simulink model "wrench_observer_R2016b"  (R2016b)
settings: Solver=VariableStepAuto  StartTime=0.0  StopTime=0.75  RelTol=1e-3
InitFcn:
  | %x_k1 = 0.00001*ones(36,1); % initialisation with initial state uncertainity
  | %P_k1 = 0.00001*ones(36); % initialisation with initial state uncertainity
values from neighbouring files (symbols this model uses):
  a_noise = 0    [parameter.m]
  alpha1 = pi/2    (= 1.57079632679)    [parameter.m]
  alpha2 = 0    [parameter.m]
  alpha3 = 0    [parameter.m]
  angular_noise = 0    [parameter.m]
  g = 9.81    [parameter.m]
  K_f_comm = 1    [parameter.m]
  K_I = [500*eye(3), zeros(3), zeros(3) ... (first row only)    [parameter.m]
  K_tau_comm = 1    [parameter.m]
  K_tau_man_comm = 1    [parameter.m]
  m = 3.9    [parameter.m]
  m_l1 = 0.3    [parameter.m]
  m_l2 = 0.35    [parameter.m]
  m_l3 = 0.35    [parameter.m]
  N_m = 1*diag([(p_noise/(3*noise_factor))^2 (p_noise/(3*noise_factor))^2 (p_noise/(3*noise_factor))^2 (a_noise/(3*noise_factor))^2 (a_noise/(3*noise_factor))^2 (a_noise/(3*noise_factor))^2 (angular_noise/(3*noise_factor))^2 (angular_noise/(3*noise_factor))^2 (angular_noise/(3*noise_factor))^2 (omega_noise/(3*noise_factor))^2 (omega_noise/(3*noise_factor))^2 (omega_noise/(3*noise_factor))^2 (theta_noise/( ...(+272 chars)    [parameter.m]
  N_p = diag(noise_factor_EKF)    [parameter.m]
  omega_dot_noise = 0    [parameter.m]
  omega_noise = 0    [parameter.m]
  p_L1_l1 = [p_L1_x_l1 p_L1_y_l1 p_L1_z_l1]'    [parameter.m]
  p_L2_l2 = [p_L2_x_l2 p_L2_y_l2 p_L2_z_l2]'    [parameter.m]
  p_L3_l3 = [p_L3_x_l3 p_L3_y_l3 p_L3_z_l3]'    [parameter.m]
  p_noise = 0    [parameter.m]
  R_B_L0 = [1 0 0;0 1 0; 0 0 1]    [parameter.m]
  T_delay = 0    [parameter.m]
  T_dis = 0.01    [parameter.m]
  theta_dot_dot_noise = 0    [parameter.m]
  theta_dot_noise = 0    [parameter.m]
  theta_noise = 0    [parameter.m]
  Ts = 1/250    (= 0.004)    [parameter.m]
  v_noise = 0    [parameter.m]
libraries: simulink x9, dspstat3 x2, dspinverses x1
(part 2 of 5)

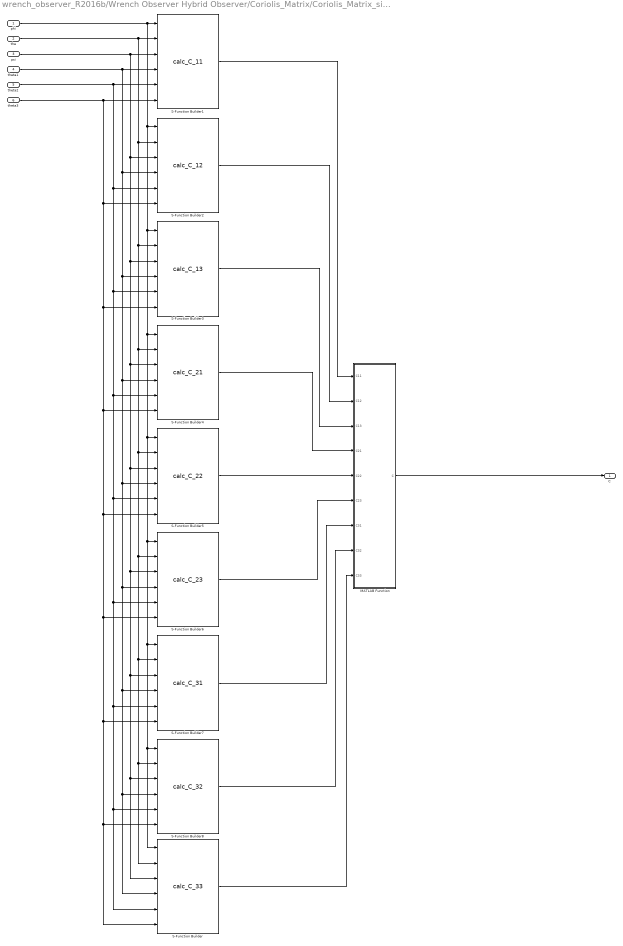
== system wrench_observer_R2016b/Wrench Observer Hybrid Observer/Coriolis_Matrix/Coriolis_Matrix_simplified ==
  phi : Inport
  the : Inport  Port=2
  psi : Inport  Port=3
  theta1 : Inport  Port=4
  theta2 : Inport  Port=5
  theta3 : Inport  Port=6
  MATLAB Function : MATLAB Function  TreatAsAtomicUnit=on
  S-Function Builder : S-Function  InitFcn=try, set_param(gcb,'FunctionName','calc_C_33'), end  FunctionName=calc_C_33  SFunctionModules=calc_C_33_wrapper C_num_simp_33 C_num_simp_33_initialize C_num_simp_33_terminate rt_nonfinite rtGetInf rtGetNaN  SFunctionDeploymentMode=off  EnableBusSupport=off  mask(S-Function Builder){}
      mask help: Simulink:masks:SFunctionBuilder_MD
      mask init: same as wrench_observer_R2016b/Motion Equations with Manipulator /Inertia_Matrix/S-Function Builder
      settings: CopyFcn=set_param(gcbh,'LinkStatus','none')  PreSaveFcn=try, set_param(gcb,'FunctionName','calc_C_33'), end  OpenFcn=sfunctionwizard(gcbh)
      mask Display: plot(val(:,1),val(:,2)),disp(sys), port_label('input',1,'phi'), port_label('input',2,'the'), port_label('input',3,'psi'), port_label('input',4,'theta1'), port_label('input',5,'theta2'), port_label('input',6,'theta3'), port_label('output',1,'C_33')
  S-Function Builder1 : S-Function  InitFcn=try, set_param(gcb,'FunctionName','calc_C_11'), end  FunctionName=calc_C_11  SFunctionModules=calc_C_11_wrapper C_num_simp_11 C_num_simp_11_initialize C_num_simp_11_terminate  SFunctionDeploymentMode=off  EnableBusSupport=off  mask(S-Function Builder){}
      mask help: Simulink:masks:SFunctionBuilder_MD
      mask init: same as wrench_observer_R2016b/Motion Equations with Manipulator /Inertia_Matrix/S-Function Builder
      settings: CopyFcn=set_param(gcbh,'LinkStatus','none')  PreSaveFcn=try, set_param(gcb,'FunctionName','calc_C_11'), end  OpenFcn=sfunctionwizard(gcbh)
      mask Display: plot(val(:,1),val(:,2)),disp(sys), port_label('input',1,'phi'), port_label('input',2,'the'), port_label('input',3,'psi'), port_label('input',4,'theta1'), port_label('input',5,'theta2'), port_label('input',6,'theta3'), port_label('output',1,'C_11')
  S-Function Builder2 : S-Function  InitFcn=try, set_param(gcb,'FunctionName','calc_C_12'), end  FunctionName=calc_C_12  SFunctionModules=calc_C_12_wrapper C_num_simp_12 C_num_simp_12_initialize C_num_simp_12_terminate  SFunctionDeploymentMode=off  EnableBusSupport=off  mask(S-Function Builder){}
      mask help: Simulink:masks:SFunctionBuilder_MD
      mask init: same as wrench_observer_R2016b/Motion Equations with Manipulator /Inertia_Matrix/S-Function Builder
      settings: CopyFcn=set_param(gcbh,'LinkStatus','none')  PreSaveFcn=try, set_param(gcb,'FunctionName','calc_C_12'), end  OpenFcn=sfunctionwizard(gcbh)
      mask Display: plot(val(:,1),val(:,2)),disp(sys), port_label('input',1,'phi'), port_label('input',2,'the'), port_label('input',3,'psi'), port_label('input',4,'theta1'), port_label('input',5,'theta2'), port_label('input',6,'theta3'), port_label('output',1,'C_12')
  S-Function Builder3 : S-Function  InitFcn=try, set_param(gcb,'FunctionName','calc_C_13'), end  FunctionName=calc_C_13  SFunctionModules=calc_C_13_wrapper C_num_simp_13 C_num_simp_13_initialize C_num_simp_13_terminate  SFunctionDeploymentMode=off  EnableBusSupport=off  mask(S-Function Builder){}
      mask help: Simulink:masks:SFunctionBuilder_MD
      mask init: same as wrench_observer_R2016b/Motion Equations with Manipulator /Inertia_Matrix/S-Function Builder
      settings: CopyFcn=set_param(gcbh,'LinkStatus','none')  PreSaveFcn=try, set_param(gcb,'FunctionName','calc_C_13'), end  OpenFcn=sfunctionwizard(gcbh)
      mask Display: plot(val(:,1),val(:,2)),disp(sys), port_label('input',1,'phi'), port_label('input',2,'the'), port_label('input',3,'psi'), port_label('input',4,'theta1'), port_label('input',5,'theta2'), port_label('input',6,'theta3'), port_label('output',1,'C_13')
  S-Function Builder4 : S-Function  InitFcn=try, set_param(gcb,'FunctionName','calc_C_21'), end  FunctionName=calc_C_21  SFunctionModules=calc_C_21_wrapper C_num_simp_21 C_num_simp_21_initialize C_num_simp_21_terminate  SFunctionDeploymentMode=off  EnableBusSupport=off  mask(S-Function Builder){}
      mask help: Simulink:masks:SFunctionBuilder_MD
      mask init: same as wrench_observer_R2016b/Motion Equations with Manipulator /Inertia_Matrix/S-Function Builder
      settings: CopyFcn=set_param(gcbh,'LinkStatus','none')  PreSaveFcn=try, set_param(gcb,'FunctionName','calc_C_21'), end  OpenFcn=sfunctionwizard(gcbh)
      mask Display: plot(val(:,1),val(:,2)),disp(sys), port_label('input',1,'phi'), port_label('input',2,'the'), port_label('input',3,'psi'), port_label('input',4,'theta1'), port_label('input',5,'theta2'), port_label('input',6,'theta3'), port_label('output',1,'C_21')
  S-Function Builder5 : S-Function  InitFcn=try, set_param(gcb,'FunctionName','calc_C_22'), end  FunctionName=calc_C_22  SFunctionModules=calc_C_22_wrapper C_num_simp_22 C_num_simp_22_initialize C_num_simp_22_terminate rt_nonfinite rtGetInf rtGetNaN  SFunctionDeploymentMode=off  EnableBusSupport=off  mask(S-Function Builder){}
      mask help: Simulink:masks:SFunctionBuilder_MD
      mask init: same as wrench_observer_R2016b/Motion Equations with Manipulator /Inertia_Matrix/S-Function Builder
      settings: CopyFcn=set_param(gcbh,'LinkStatus','none')  PreSaveFcn=try, set_param(gcb,'FunctionName','calc_C_22'), end  OpenFcn=sfunctionwizard(gcbh)
      mask Display: plot(val(:,1),val(:,2)),disp(sys), port_label('input',1,'phi'), port_label('input',2,'the'), port_label('input',3,'psi'), port_label('input',4,'theta1'), port_label('input',5,'theta2'), port_label('input',6,'theta3'), port_label('output',1,'C_22')
  S-Function Builder6 : S-Function  InitFcn=try, set_param(gcb,'FunctionName','calc_C_23'), end  FunctionName=calc_C_23  SFunctionModules=calc_C_23_wrapper C_num_simp_23 C_num_simp_23_initialize C_num_simp_23_terminate rt_nonfinite rtGetInf rtGetNaN  SFunctionDeploymentMode=off  EnableBusSupport=off  mask(S-Function Builder){}
      mask help: Simulink:masks:SFunctionBuilder_MD
      mask init: same as wrench_observer_R2016b/Motion Equations with Manipulator /Inertia_Matrix/S-Function Builder
      settings: CopyFcn=set_param(gcbh,'LinkStatus','none')  PreSaveFcn=try, set_param(gcb,'FunctionName','calc_C_23'), end  OpenFcn=sfunctionwizard(gcbh)
      mask Display: plot(val(:,1),val(:,2)),disp(sys), port_label('input',1,'phi'), port_label('input',2,'the'), port_label('input',3,'psi'), port_label('input',4,'theta1'), port_label('input',5,'theta2'), port_label('input',6,'theta3'), port_label('output',1,'C_23')
  S-Function Builder7 : S-Function  InitFcn=try, set_param(gcb,'FunctionName','calc_C_31'), end  FunctionName=calc_C_31  SFunctionModules=calc_C_31_wrapper C_num_simp_31 C_num_simp_31_initialize C_num_simp_31_terminate  SFunctionDeploymentMode=off  EnableBusSupport=off  mask(S-Function Builder){}
      mask help: Simulink:masks:SFunctionBuilder_MD
      mask init: same as wrench_observer_R2016b/Motion Equations with Manipulator /Inertia_Matrix/S-Function Builder
      settings: CopyFcn=set_param(gcbh,'LinkStatus','none')  PreSaveFcn=try, set_param(gcb,'FunctionName','calc_C_31'), end  OpenFcn=sfunctionwizard(gcbh)
      mask Display: plot(val(:,1),val(:,2)),disp(sys), port_label('input',1,'phi'), port_label('input',2,'the'), port_label('input',3,'psi'), port_label('input',4,'theta1'), port_label('input',5,'theta2'), port_label('input',6,'theta3'), port_label('output',1,'C_31')
  S-Function Builder8 : S-Function  InitFcn=try, set_param(gcb,'FunctionName','calc_C_32'), end  FunctionName=calc_C_32  SFunctionModules=calc_C_32_wrapper C_num_simp_32 C_num_simp_32_initialize C_num_simp_32_terminate rt_nonfinite rtGetInf rtGetNaN  SFunctionDeploymentMode=off  EnableBusSupport=off  mask(S-Function Builder){}
      mask help: Simulink:masks:SFunctionBuilder_MD
      mask init: same as wrench_observer_R2016b/Motion Equations with Manipulator /Inertia_Matrix/S-Function Builder
      settings: CopyFcn=set_param(gcbh,'LinkStatus','none')  PreSaveFcn=try, set_param(gcb,'FunctionName','calc_C_32'), end  OpenFcn=sfunctionwizard(gcbh)
      mask Display: plot(val(:,1),val(:,2)),disp(sys), port_label('input',1,'phi'), port_label('input',2,'the'), port_label('input',3,'psi'), port_label('input',4,'theta1'), port_label('input',5,'theta2'), port_label('input',6,'theta3'), port_label('output',1,'C_32')
  C : Outport
  wires:
  S-Function Builder5/1 -> MATLAB Function/5(C22)
  theta2/1 -> S-Function Builder2/5, S-Function Builder3/5, S-Function Builder4/5, S-Function Builder5/5, S-Function Builder6/5, S-Function Builder7/5, S-Function Builder8/5, S-Function Builder/5, S-Function Builder1/5
  S-Function Builder3/1 -> MATLAB Function/3(C13)
  theta1/1 -> S-Function Builder2/4, S-Function Builder3/4, S-Function Builder4/4, S-Function Builder5/4, S-Function Builder6/4, S-Function Builder7/4, S-Function Builder8/4, S-Function Builder/4, S-Function Builder1/4
  theta3/1 -> S-Function Builder2/6, S-Function Builder3/6, S-Function Builder4/6, S-Function Builder5/6, S-Function Builder6/6, S-Function Builder7/6, S-Function Builder8/6, S-Function Builder/6, S-Function Builder1/6
  psi/1 -> S-Function Builder1/3, S-Function Builder2/3, S-Function Builder3/3, S-Function Builder4/3, S-Function Builder5/3, S-Function Builder6/3, S-Function Builder7/3, S-Function Builder8/3, S-Function Builder/3
  phi/1 -> S-Function Builder2/1, S-Function Builder3/1, S-Function Builder4/1, S-Function Builder5/1, S-Function Builder6/1, S-Function Builder7/1, S-Function Builder8/1, S-Function Builder/1, S-Function Builder1/1
  the/1 -> S-Function Builder2/2, S-Function Builder3/2, S-Function Builder4/2, S-Function Builder5/2, S-Function Builder6/2, S-Function Builder7/2, S-Function Builder8/2, S-Function Builder/2, S-Function Builder1/2
  S-Function Builder2/1 -> MATLAB Function/2(C12)
  S-Function Builder/1 -> MATLAB Function/9(C33)
  S-Function Builder7/1 -> MATLAB Function/7(C31)
  S-Function Builder1/1 -> MATLAB Function/1(C11)
  S-Function Builder8/1 -> MATLAB Function/8(C32)
  S-Function Builder6/1 -> MATLAB Function/6(C23)
  S-Function Builder4/1 -> MATLAB Function/4(C21)
  MATLAB Function/1(C) -> C/1

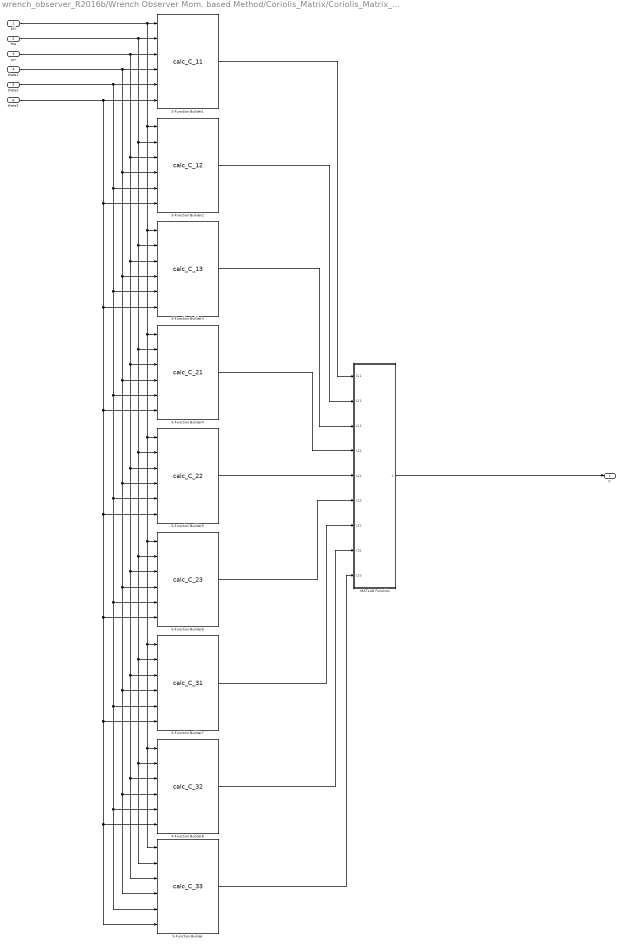
== system wrench_observer_R2016b/Wrench Observer Mom. based Method/Coriolis_Matrix/Coriolis_Matrix_simplified ==
  phi : Inport
  the : Inport  Port=2
  psi : Inport  Port=3
  theta1 : Inport  Port=4
  theta2 : Inport  Port=5
  theta3 : Inport  Port=6
  MATLAB Function : MATLAB Function  TreatAsAtomicUnit=on
  S-Function Builder : S-Function  InitFcn=try, set_param(gcb,'FunctionName','calc_C_33'), end  FunctionName=calc_C_33  SFunctionModules=calc_C_33_wrapper C_num_simp_33 C_num_simp_33_initialize C_num_simp_33_terminate rt_nonfinite rtGetInf rtGetNaN  SFunctionDeploymentMode=off  EnableBusSupport=off  mask(S-Function Builder){}
      mask help: Simulink:masks:SFunctionBuilder_MD
      mask init: same as wrench_observer_R2016b/Motion Equations with Manipulator /Inertia_Matrix/S-Function Builder
      settings: CopyFcn=set_param(gcbh,'LinkStatus','none')  PreSaveFcn=try, set_param(gcb,'FunctionName','calc_C_33'), end  OpenFcn=sfunctionwizard(gcbh)
      mask Display: plot(val(:,1),val(:,2)),disp(sys), port_label('input',1,'phi'), port_label('input',2,'the'), port_label('input',3,'psi'), port_label('input',4,'theta1'), port_label('input',5,'theta2'), port_label('input',6,'theta3'), port_label('output',1,'C_33')
  S-Function Builder1 : S-Function  InitFcn=try, set_param(gcb,'FunctionName','calc_C_11'), end  FunctionName=calc_C_11  SFunctionModules=calc_C_11_wrapper C_num_simp_11 C_num_simp_11_initialize C_num_simp_11_terminate  SFunctionDeploymentMode=off  EnableBusSupport=off  mask(S-Function Builder){}
      mask help: Simulink:masks:SFunctionBuilder_MD
      mask init: same as wrench_observer_R2016b/Motion Equations with Manipulator /Inertia_Matrix/S-Function Builder
      settings: CopyFcn=set_param(gcbh,'LinkStatus','none')  PreSaveFcn=try, set_param(gcb,'FunctionName','calc_C_11'), end  OpenFcn=sfunctionwizard(gcbh)
      mask Display: plot(val(:,1),val(:,2)),disp(sys), port_label('input',1,'phi'), port_label('input',2,'the'), port_label('input',3,'psi'), port_label('input',4,'theta1'), port_label('input',5,'theta2'), port_label('input',6,'theta3'), port_label('output',1,'C_11')
  S-Function Builder2 : S-Function  InitFcn=try, set_param(gcb,'FunctionName','calc_C_12'), end  FunctionName=calc_C_12  SFunctionModules=calc_C_12_wrapper C_num_simp_12 C_num_simp_12_initialize C_num_simp_12_terminate  SFunctionDeploymentMode=off  EnableBusSupport=off  mask(S-Function Builder){}
      mask help: Simulink:masks:SFunctionBuilder_MD
      mask init: same as wrench_observer_R2016b/Motion Equations with Manipulator /Inertia_Matrix/S-Function Builder
      settings: CopyFcn=set_param(gcbh,'LinkStatus','none')  PreSaveFcn=try, set_param(gcb,'FunctionName','calc_C_12'), end  OpenFcn=sfunctionwizard(gcbh)
      mask Display: plot(val(:,1),val(:,2)),disp(sys), port_label('input',1,'phi'), port_label('input',2,'the'), port_label('input',3,'psi'), port_label('input',4,'theta1'), port_label('input',5,'theta2'), port_label('input',6,'theta3'), port_label('output',1,'C_12')
  S-Function Builder3 : S-Function  InitFcn=try, set_param(gcb,'FunctionName','calc_C_13'), end  FunctionName=calc_C_13  SFunctionModules=calc_C_13_wrapper C_num_simp_13 C_num_simp_13_initialize C_num_simp_13_terminate  SFunctionDeploymentMode=off  EnableBusSupport=off  mask(S-Function Builder){}
      mask help: Simulink:masks:SFunctionBuilder_MD
      mask init: same as wrench_observer_R2016b/Motion Equations with Manipulator /Inertia_Matrix/S-Function Builder
      settings: CopyFcn=set_param(gcbh,'LinkStatus','none')  PreSaveFcn=try, set_param(gcb,'FunctionName','calc_C_13'), end  OpenFcn=sfunctionwizard(gcbh)
      mask Display: plot(val(:,1),val(:,2)),disp(sys), port_label('input',1,'phi'), port_label('input',2,'the'), port_label('input',3,'psi'), port_label('input',4,'theta1'), port_label('input',5,'theta2'), port_label('input',6,'theta3'), port_label('output',1,'C_13')
  S-Function Builder4 : S-Function  InitFcn=try, set_param(gcb,'FunctionName','calc_C_21'), end  FunctionName=calc_C_21  SFunctionModules=calc_C_21_wrapper C_num_simp_21 C_num_simp_21_initialize C_num_simp_21_terminate  SFunctionDeploymentMode=off  EnableBusSupport=off  mask(S-Function Builder){}
      mask help: Simulink:masks:SFunctionBuilder_MD
      mask init: same as wrench_observer_R2016b/Motion Equations with Manipulator /Inertia_Matrix/S-Function Builder
      settings: CopyFcn=set_param(gcbh,'LinkStatus','none')  PreSaveFcn=try, set_param(gcb,'FunctionName','calc_C_21'), end  OpenFcn=sfunctionwizard(gcbh)
      mask Display: plot(val(:,1),val(:,2)),disp(sys), port_label('input',1,'phi'), port_label('input',2,'the'), port_label('input',3,'psi'), port_label('input',4,'theta1'), port_label('input',5,'theta2'), port_label('input',6,'theta3'), port_label('output',1,'C_21')
  S-Function Builder5 : S-Function  InitFcn=try, set_param(gcb,'FunctionName','calc_C_22'), end  FunctionName=calc_C_22  SFunctionModules=calc_C_22_wrapper C_num_simp_22 C_num_simp_22_initialize C_num_simp_22_terminate rt_nonfinite rtGetInf rtGetNaN  SFunctionDeploymentMode=off  EnableBusSupport=off  mask(S-Function Builder){}
      mask help: Simulink:masks:SFunctionBuilder_MD
      mask init: same as wrench_observer_R2016b/Motion Equations with Manipulator /Inertia_Matrix/S-Function Builder
      settings: CopyFcn=set_param(gcbh,'LinkStatus','none')  PreSaveFcn=try, set_param(gcb,'FunctionName','calc_C_22'), end  OpenFcn=sfunctionwizard(gcbh)
      mask Display: plot(val(:,1),val(:,2)),disp(sys), port_label('input',1,'phi'), port_label('input',2,'the'), port_label('input',3,'psi'), port_label('input',4,'theta1'), port_label('input',5,'theta2'), port_label('input',6,'theta3'), port_label('output',1,'C_22')
  S-Function Builder6 : S-Function  InitFcn=try, set_param(gcb,'FunctionName','calc_C_23'), end  FunctionName=calc_C_23  SFunctionModules=calc_C_23_wrapper C_num_simp_23 C_num_simp_23_initialize C_num_simp_23_terminate rt_nonfinite rtGetInf rtGetNaN  SFunctionDeploymentMode=off  EnableBusSupport=off  mask(S-Function Builder){}
      mask help: Simulink:masks:SFunctionBuilder_MD
      mask init: same as wrench_observer_R2016b/Motion Equations with Manipulator /Inertia_Matrix/S-Function Builder
      settings: CopyFcn=set_param(gcbh,'LinkStatus','none')  PreSaveFcn=try, set_param(gcb,'FunctionName','calc_C_23'), end  OpenFcn=sfunctionwizard(gcbh)
      mask Display: plot(val(:,1),val(:,2)),disp(sys), port_label('input',1,'phi'), port_label('input',2,'the'), port_label('input',3,'psi'), port_label('input',4,'theta1'), port_label('input',5,'theta2'), port_label('input',6,'theta3'), port_label('output',1,'C_23')
  S-Function Builder7 : S-Function  InitFcn=try, set_param(gcb,'FunctionName','calc_C_31'), end  FunctionName=calc_C_31  SFunctionModules=calc_C_31_wrapper C_num_simp_31 C_num_simp_31_initialize C_num_simp_31_terminate  SFunctionDeploymentMode=off  EnableBusSupport=off  mask(S-Function Builder){}
      mask help: Simulink:masks:SFunctionBuilder_MD
      mask init: same as wrench_observer_R2016b/Motion Equations with Manipulator /Inertia_Matrix/S-Function Builder
      settings: CopyFcn=set_param(gcbh,'LinkStatus','none')  PreSaveFcn=try, set_param(gcb,'FunctionName','calc_C_31'), end  OpenFcn=sfunctionwizard(gcbh)
      mask Display: plot(val(:,1),val(:,2)),disp(sys), port_label('input',1,'phi'), port_label('input',2,'the'), port_label('input',3,'psi'), port_label('input',4,'theta1'), port_label('input',5,'theta2'), port_label('input',6,'theta3'), port_label('output',1,'C_31')
  S-Function Builder8 : S-Function  InitFcn=try, set_param(gcb,'FunctionName','calc_C_32'), end  FunctionName=calc_C_32  SFunctionModules=calc_C_32_wrapper C_num_simp_32 C_num_simp_32_initialize C_num_simp_32_terminate rt_nonfinite rtGetInf rtGetNaN  SFunctionDeploymentMode=off  EnableBusSupport=off  mask(S-Function Builder){}
      mask help: Simulink:masks:SFunctionBuilder_MD
      mask init: same as wrench_observer_R2016b/Motion Equations with Manipulator /Inertia_Matrix/S-Function Builder
      settings: CopyFcn=set_param(gcbh,'LinkStatus','none')  PreSaveFcn=try, set_param(gcb,'FunctionName','calc_C_32'), end  OpenFcn=sfunctionwizard(gcbh)
      mask Display: plot(val(:,1),val(:,2)),disp(sys), port_label('input',1,'phi'), port_label('input',2,'the'), port_label('input',3,'psi'), port_label('input',4,'theta1'), port_label('input',5,'theta2'), port_label('input',6,'theta3'), port_label('output',1,'C_32')
  C : Outport
  wires:
  S-Function Builder5/1 -> MATLAB Function/5(C22)
  theta2/1 -> S-Function Builder2/5, S-Function Builder3/5, S-Function Builder4/5, S-Function Builder5/5, S-Function Builder6/5, S-Function Builder7/5, S-Function Builder8/5, S-Function Builder/5, S-Function Builder1/5
  S-Function Builder3/1 -> MATLAB Function/3(C13)
  theta1/1 -> S-Function Builder2/4, S-Function Builder3/4, S-Function Builder4/4, S-Function Builder5/4, S-Function Builder6/4, S-Function Builder7/4, S-Function Builder8/4, S-Function Builder/4, S-Function Builder1/4
  theta3/1 -> S-Function Builder2/6, S-Function Builder3/6, S-Function Builder4/6, S-Function Builder5/6, S-Function Builder6/6, S-Function Builder7/6, S-Function Builder8/6, S-Function Builder/6, S-Function Builder1/6
  psi/1 -> S-Function Builder1/3, S-Function Builder2/3, S-Function Builder3/3, S-Function Builder4/3, S-Function Builder5/3, S-Function Builder6/3, S-Function Builder7/3, S-Function Builder8/3, S-Function Builder/3
  phi/1 -> S-Function Builder2/1, S-Function Builder3/1, S-Function Builder4/1, S-Function Builder5/1, S-Function Builder6/1, S-Function Builder7/1, S-Function Builder8/1, S-Function Builder/1, S-Function Builder1/1
  the/1 -> S-Function Builder2/2, S-Function Builder3/2, S-Function Builder4/2, S-Function Builder5/2, S-Function Builder6/2, S-Function Builder7/2, S-Function Builder8/2, S-Function Builder/2, S-Function Builder1/2
  S-Function Builder2/1 -> MATLAB Function/2(C12)
  S-Function Builder/1 -> MATLAB Function/9(C33)
  S-Function Builder7/1 -> MATLAB Function/7(C31)
  S-Function Builder1/1 -> MATLAB Function/1(C11)
  S-Function Builder8/1 -> MATLAB Function/8(C32)
  S-Function Builder6/1 -> MATLAB Function/6(C23)
  S-Function Builder4/1 -> MATLAB Function/4(C21)
  MATLAB Function/1(C) -> C/1

== matlab function wrench_observer_R2016b/Wrench Observer Mom. based Method/MATLAB Function2 ==
  data: q_meas input; G_est output; alpha1 parameter; alpha2 parameter; alpha3 parameter; R_B_L0 parameter; g parameter; m parameter; m_l2 parameter; m_l3 parameter; m_l1 parameter; p_L1_l1 parameter; p_L2_l2 parameter; p_L3_l3 parameter
function G_est = Gravity_Matrix(q_meas, alpha1, alpha2, alpha3, R_B_L0, g, m, m_l2, m_l3, m_l1, p_L1_l1, p_L2_l2, p_L3_l3)
phi_E = q_meas(4);
theta_E = q_meas(5);
psi_E = q_meas(6);
theta1 = q_meas(7);
theta2 = q_meas(8);
theta3 = q_meas(9);
% theta4 = q(10);
% theta5 = q(11);

sphi = sin(phi_E); cphi = cos(phi_E);
sth = sin(theta_E); cth = cos(theta_E);
spsi = sin(psi_E); cpsi = cos(psi_E);
sth1 = sin(theta1); cth1 = cos(theta1); sth2 = sin(theta2); cth2 = cos(theta2); sth3 = sin(theta3); cth3 = cos(theta3);
salp1 = sin(alpha1); calp1 = cos(alpha1); salp2 = sin(alpha2); calp2 = cos(alpha2); salp3 = sin(alpha3); calp3 = cos(alpha3);

p_L1_x_l1 = p_L1_l1(1); p_L1_y_l1 = p_L1_l1(2); p_L1_z_l1 = p_L1_l1(3);
p_L2_x_l2 = p_L2_l2(1); p_L2_y_l2 = p_L2_l2(2); p_L2_z_l2 = p_L2_l2(3);
p_L3_x_l3 = p_L3_l3(1); p_L3_y_l3 = p_L3_l3(2); p_L3_z_l3 = p_L3_l3(3);
%% Rotation matrix from inertial to body frame
R_IB = [cpsi*cth cpsi*sth*sphi-spsi*cphi cpsi*sth*cphi+spsi*sphi;
        spsi*cth spsi*sth*sphi+cpsi*cphi spsi*sth*cphi-cpsi*sphi;
        -sth cth*sphi cth*cphi];

%% Rotation matrices from link i to manipulator base {L0}
% R_th_1 = [cth1 -sth1 0 0;
%     sth1 cth1 0 0;
%     0 0 1 0;
%     0 0 0 1];
% R_alpha_1 = [1 0 0 0;
%     0 calp1 -salp1 0;
%     0 salp1 calp1 0;
%     0 0 0 1];
% R_th_2 = [cth2 -sth2 0 0;
%     sth2 cth2 0 0;
%     0 0 1 0;
%     0 0 0 1];
% R_alpha_2 = [1 0 0 0;
%     0 calp2 -salp2 0;
%     0 salp2 calp2 0;
%     0 0 0 1];
% R_th_3 = [cth3 -sth3 0 0;
%     sth3 cth3 0 0;
%     0 0 1 0;
%     0 0 0 1];
% R_alpha_3 = [1 0 0 0;
%     0 calp3 -salp3 0;
%     0 salp3 calp3 0;
%     0 0 0 1];
% R_th_4 = [cth4 -sth4 0 0;
%         sth4 cth4 0 0;
%         0 0 1 0;
%         0 0 0 1];
% R_alpha_4 = [1 0 0 0;
%            0 calph4 -salph4 0;
%            0 salph4 calph4 0;
%            0 0 0 1];
% R_th_5 = [cth5 -sth5 0 0;
%         sth5 cth5 0 0;
%         0 0 1 0;
%         0 0 0 1];
% R_alpha_5 = [1 0 0 0;
%            0 calph5 -salph5 0;
%            0 salph5 calph5 0;
%            0 0 0 1];

% transformation matrices from link i to link i-1
% T_L0_L1 = R_th_1 * [1 0 0 0;0 1 0 0;0 0 1 d1;0 0 0 0] * [1 0 0 a1;0 1 0 0;0 0 1 0;0 0 0 1] * R_alpha_1;
% T_L1_L2 = R_th_2 * [1 0 0 0;0 1 0 0;0 0 1 d2;0 0 0 0] * [1 0 0 a2;0 1 0 0;0 0 1 0;0 0 0 1] * R_alpha_2;
% T_L2_L3 = R_th_3 * [1 0 0 0;0 1 0 0;0 0 1 d3;0 0 0 0] * [1 0 0 a3;0 1 0 0;0 0 1 0;0 0 0 1] * R_alpha_3;
% T_L3_L4 = R_th_4 * [1 0 0 0;0 1 0 0;0 0 1 d4;0 0 0 0] * [1 0 0 a4;0 1 0 0;0 0 1 0;0 0 0 1] * R_alpha_4;
% T_L4_L5 = R_th_5 * [1 0 0 0;0 1 0 0;0 0 1 d5;0 0 0 0] * [1 0 0 a5;0 1 0 0;0 0 1 0;0 0 0 1] * R_alpha_5;

% transformatin matrices from link i to manipulator base {L0}
% T_L0_L2 = T_L0_L1*T_L1_L2;
% T_L0_L3 = T_L0_L2*T_L2_L3;
% T_L0_L4 = T_L0_L3*T_L3_L4;
% T_L0_L5 = T_L0_L4*T_L4_L5;

% rotation matrices from link i to manipulator base {L0}
% R_L0_L1 = T_L0_L1(1:3,1:3);
% R_L0_L2 = T_L0_L2(1:3,1:3);
% R_L0_L3 = T_L0_L3(1:3,1:3);
% R_L0_L4 = T_L0_L4(1:3,1:3);
% R_L0_L5 = T_L0_L5(1:3,1:3);

R_L0_L1 = [ cth1, -calp1*sth1,  sth1*salp1;
            sth1,  cth1*calp1, -cth1*salp1;
             0,         salp1,       calp1];

R_L0_L2 = [ cth1*cth2 - calp1*sth1*sth2, sth1*salp1*salp2 - cth1*calp2*sth2 - cth2*calp1*calp2*sth1, cth1*sth2*salp2 + calp2*sth1*salp1 + cth2*calp1*sth1*salp2;
            cth2*sth1 + cth1*calp1*sth2, cth1*cth2*calp1*calp2 - cth1*salp1*salp2 - calp2*sth1*sth2, sth1*sth2*salp2 - cth1*calp2*salp1 - cth1*cth2*calp1*salp2;
             sth2*salp1,                                                   calp1*salp2 + cth2*calp2*salp1,                       calp1*calp2 - cth2*salp1*salp2];
         
R_L0_L3 = [ cth3*(cth1*cth2 - calp1*sth1*sth2) - sth3*(calp2*cth1*sth2 - salp1*salp2*sth1 + calp1*calp2*cth2*sth1),   salp3*(calp2*salp1*sth1 + salp2*cth1*sth2 + calp1*salp2*cth2*sth1) - calp3*cth3*(calp2*cth1*sth2 - salp1*salp2*sth1 + calp1*calp2*cth2*sth1) - calp3*sth3*(cth1*cth2 - calp1*sth1*sth2), calp3*(calp2*salp1*sth1 + salp2*cth1*sth2 + calp1*salp2*cth2*sth1) + salp3*cth3*(calp2*cth1*sth2 - salp1*salp2*sth1 + calp1*calp2*cth2*sth1) + salp3*sth3*(cth1*cth2 - calp1*sth1*sth2);
            cth3*(cth2*sth1 + calp1*cth1*sth2) - sth3*(salp1*salp2*cth1 + calp2*sth1*sth2 - calp1*calp2*cth1*cth2), - salp3*(calp2*salp1*cth1 - salp2*sth1*sth2 + calp1*salp2*cth1*cth2) - calp3*cth3*(salp1*salp2*cth1 + calp2*sth1*sth2 - calp1*calp2*cth1*cth2) - calp3*sth3*(cth2*sth1 + calp1*cth1*sth2), salp3*cth3*(salp1*salp2*cth1 + calp2*sth1*sth2 - calp1*calp2*cth1*cth2) - calp3*(calp2*salp1*cth1 - salp2*sth1*sth2 + calp1*salp2*cth1*cth2) + salp3*sth3*(cth2*sth1 + calp1*cth1*sth2);
             sth3*(calp1*salp2 + calp2*salp1*cth2) + salp1*cth3*sth2,                                                                                                                                      salp3*(calp1*calp2 - salp1*salp2*cth2) + calp3*cth3*(calp1*salp2 + calp2*salp1*cth2) - calp3*salp1*sth2*sth3,                                                                 calp3*(calp1*calp2 - salp1*salp2*cth2) - salp3*cth3*(calp1*salp2 + calp2*salp1*cth2) + salp1*salp3*sth2*sth3];

%% Gravity vector
a = R_B_L0(1,1)*R_IB(3,1)+ R_B_L0(2,1)*R_IB(3,2)+ R_B_L0(3,1)*R_IB(3,3);
b = R_B_L0(1,2)*R_IB(3,1)+ R_B_L0(2,2)*R_IB(3,2)+ R_B_L0(3,2)*R_IB(3,3);
c = R_B_L0(1,3)*R_IB(3,1)+ R_B_L0(2,3)*R_IB(3,2)+ R_B_L0(3,3)*R_IB(3,3);
% partial derivatives
dadphi = -R_B_L0(2,1)*cphi*cth + R_B_L0(3,1)*sphi*cth;
dadth = R_B_L0(1,1)*cth + R_B_L0(2,1)*sphi*sth + R_B_L0(3,1)*cphi*sth;
dadpsi = 0;
dbdphi = -R_B_L0(2,2)*cphi*cth + R_B_L0(3,2)*sphi*cth;
dbdth = R_B_L0(1,2)*cth + R_B_L0(2,2)*sphi*sth + R_B_L0(3,2)*cphi*sth;
dbdpsi = 0;
dcdphi = -R_B_L0(2,3)*cphi*cth + R_B_L0(3,3)*sphi*cth;
dcdth = R_B_L0(1,3)*cth + R_B_L0(2,3)*sphi*sth + R_B_L0(3,3)*cphi*sth;
dcdpsi = 0;

% gravity vector UAV
dUuav = [0 0 g*m 0 0 0 0 0 0]';
% gravity vector link 1
dUman_1 = zeros(9,1);
dUman_1(1) = 0; dUman_1(2) = 0; dUman_1(3) = g*m_l1;
dUman_1(4) = p_L1_x_l1*m_l1*g*(R_L0_L1(1,1)*dadphi + R_L0_L1(2,1)*dbdphi + R_L0_L1(3,1)*dcdphi)                                       + p_L1_y_l1*m_l1*g*(R_L0_L1(1,2)*dadphi + R_L0_L1(2,2)*dbdphi + R_L0_L1(3,2)*dcdphi)      + p_L1_z_l1*m_l1*g*(R_L0_L1(1,3)*dadphi + R_L0_L1(2,3)*dbdphi + R_L0_L1(3,3)*dcdphi);
dUman_1(5) = p_L1_x_l1*m_l1*g*(R_L0_L1(1,1)*dadth + R_L0_L1(2,1)*dbdth + R_L0_L1(3,1)*dcdth)                                          + p_L1_y_l1*m_l1*g*(R_L0_L1(1,2)*dadth + R_L0_L1(2,2)*dbdth + R_L0_L1(3,2)*dcdth)         + p_L1_z_l1*m_l1*g*(R_L0_L1(1,3)*dadth + R_L0_L1(2,3)*dbdth + R_L0_L1(3,3)*dcdth);
dUman_1(6) = p_L1_x_l1*m_l1*g*(R_L0_L1(1,1)*dadpsi + R_L0_L1(2,1)*dbdpsi + R_L0_L1(3,1)*dcdpsi)                                       + p_L1_y_l1*m_l1*g*(R_L0_L1(1,2)*dadpsi + R_L0_L1(2,2)*dbdpsi + R_L0_L1(3,2)*dcdpsi)      + p_L1_z_l1*m_l1*g*(R_L0_L1(1,3)*dadpsi + R_L0_L1(2,3)*dbdpsi + R_L0_L1(3,3)*dcdpsi);
dUman_1(7) = p_L1_x_l1*m_l1*g*(sth1*a - cth1*b)                                                                                       + p_L1_y_l1*m_l1*g*(-cth1*calp1*a + sth1*calp1*b)                                         + p_L1_z_l1*m_l1*g*(cth1*salp1*a + sth1*salp1*b);
dUman_1(8) = 0;
dUman_1(9) = 0;
% gravity vector link 2
dUman_2 = zeros(9,1);
dUman_2(1) = 0; dUman_2(2) = 0; dUman_2(3) = g*m_l2;
dUman_2(4) = p_L2_x_l2*m_l2*g*(R_L0_L2(1,1)*dadphi + R_L0_L2(2,1)*dbdphi + R_L0_L2(3,1)*dcdphi)                                       + p_L2_y_l2*m_l2*g*(R_L0_L2(1,2)*dadphi + R_L0_L2(2,2)*dbdphi + R_L0_L2(3,2)*dcdphi)                                                                  + p_L2_z_l2*m_l2*g*(R_L0_L2(1,3)*dadphi + R_L0_L2(2,3)*dbdphi + R_L0_L2(3,3)*dcdphi);
dUman_2(5) = p_L2_x_l2*m_l2*g*(R_L0_L2(1,1)*dadth + R_L0_L2(2,1)*dbdth + R_L0_L2(3,1)*dcdth)                                          + p_L2_y_l2*m_l2*g*(R_L0_L2(1,2)*dadth + R_L0_L2(2,2)*dbdth + R_L0_L2(3,2)*dcdth)                                                                     + p_L2_z_l2*m_l2*g*(R_L0_L2(1,3)*dadth + R_L0_L2(2,3)*dbdth + R_L0_L2(3,3)*dcdth);
dUman_2(6) = p_L2_x_l2*m_l2*g*(R_L0_L2(1,1)*dadpsi + R_L0_L2(2,1)*dbdpsi + R_L0_L2(3,1)*dcdpsi)                                       + p_L2_y_l2*m_l2*g*(R_L0_L2(1,2)*dadpsi + R_L0_L2(2,2)*dbdpsi + R_L0_L2(3,2)*dcdpsi)                                                                  + p_L2_z_l2*m_l2*g*(R_L0_L2(1,3)*dadpsi + R_L0_L2(2,3)*dbdpsi + R_L0_L2(3,3)*dcdpsi);
dUman_2(7) = p_L2_x_l2*m_l2*g*((sth1*cth2+cth1*sth2*calp1)*a + (-cth1*cth2+sth1*sth2*calp1)*b)                                        + p_L2_y_l2*m_l2*g*((-cth1*salp1*salp2-sth1*sth2*calp2+cth1*cth2*calp1*calp2)*a + (sth1*cth2*calp1*calp2-sth1*salp1*salp2+cth1*sth2*calp2)*b)         + p_L2_z_l2*m_l2*g*((sth1*sth2*salp2-cth2*salp1*calp2-cth1*cth2*calp1*salp2)*a + (-cth1*sth2*salp2-sth1*salp1*calp2-sth1*cth2*calp1*salp2)*b);
dUman_2(8) = p_L2_x_l2*m_l2*g*((sth2*cth1+cth2*sth1*calp1)*a + (sth2*sth1-cth2*cth1*calp1)*b + (-cth2*salp1)*c)                       + p_L2_y_l2*m_l2*g*((cth2*cth1*calp2-sth2*sth1*calp1*calp2)*a + (sth2*cth1*calp1*calp2+cth2*sth1*calp2)*b + (sth2*salp1*calp2)*c)                     + p_L2_z_l2*m_l2*g*((-cth2*cth1*salp2+sth2*sth1*calp1*salp2)*a + (-cth2*sth1*salp2)*b + (-sth2*salp1*salp2)*c);
dUman_2(9) = 0;
% gravity vector link 3
dUman_3 = zeros(9,1);
dUman_3(1) = 0; dUman_3(2) = 0; dUman_3(3) = g*m_l3;
dUman_3(4) = p_L3_x_l3*m_l3*g*(R_L0_L3(1,1)*dadphi + R_L0_L3(2,1)*dbdphi + R_L0_L3(3,1)*dcdphi)                                                                                                                                                                                                         + p_L3_y_l3*m_l3*g*(R_L0_L3(1,2)*dadphi + R_L0_L3(2,2)*dbdphi + R_L0_L3(3,2)*dcdphi)                                                                                                                                                                                                                                                                                            + p_L3_z_l3*m_l3*g*(R_L0_L3(1,3)*dadphi + R_L0_L3(2,3)*dbdphi + R_L0_L3(3,3)*dcdphi);
dUman_3(5) = p_L3_x_l3*m_l3*g*(R_L0_L3(1,1)*dadth + R_L0_L3(2,1)*dbdth + R_L0_L3(3,1)*dcdth)                                                                                                                                                                                                            + p_L3_y_l3*m_l3*g*(R_L0_L3(1,2)*dadth + R_L0_L3(2,2)*dbdth + R_L0_L3(3,2)*dcdth)                                                                                                                                                                                                                                                                                               + p_L3_z_l3*m_l3*g*(R_L0_L3(1,3)*dadth + R_L0_L3(2,3)*dbdth + R_L0_L3(3,3)*dcdth);
dUman_3(6) = p_L3_x_l3*m_l3*g*(R_L0_L3(1,1)*dadpsi + R_L0_L3(2,1)*dbdpsi + R_L0_L3(3,1)*dcdpsi)                                                                                                                                                                                                         + p_L3_y_l3*m_l3*g*(R_L0_L3(1,2)*dadpsi + R_L0_L3(2,2)*dbdpsi + R_L0_L3(3,2)*dcdpsi)                                                                                                                                                                                                                                                                                            + p_L3_z_l3*m_l3*g*(R_L0_L3(1,3)*dadpsi + R_L0_L3(2,3)*dbdpsi + R_L0_L3(3,3)*dcdpsi);
dUman_3(7) = p_L3_x_l3*m_l3*g*((sth1*cth2*cth3+cth1*sth2*calp1-sth1*sth2*sth3*calp2+cth1*salp1*salp2-cth1*cth2*calp1*calp2)*a + (cth1*cth2*cth3+cth1*sth2*calp1+cth1*sth2*sth3*calp2-sth1*salp1*salp2-sth1*cth2*calp1*calp2)*b)                                                                         + p_L3_y_l3*m_l3*g*((sth1*sth2*salp2*salp3-cth1*salp1*calp2-cth1*cth2*calp1*calp2-sth1*sth2*cth3*calp2*calp3+cth1*salp1*salp2-cth1*cth2*calp1*calp2-sth1*cth2*sth3*calp3+cth1*sth2*calp1)*a + (-sth1*salp1*calp2*salp3+cth1*sth2*salp2+sth1*cth2*calp1*salp2+cth1*sth2*cth3*calp2*calp3+sth1*salp1*salp2-sth1*cth2*calp1*calp2+cth1*cth2*sth3*calp3+sth1*sth2*calp1)*b)         + p_L3_z_l3*m_l3*g*((sth1*sth2*salp2*calp3-cth1*salp1*calp2-cth1*cth2*calp1*salp2+sth1*sth2*cth3*calp2*salp3+cth1*salp1*salp2-cth1*cth2*calp1*calp2+sth1*cth2*sth3*salp3+cth1*sth2*calp1)*a + (-cth1*sth2*cth3*calp2*salp3+sth1*salp1*salp2-sth1*cth2*calp1*calp2-sth1*salp1*calp2*calp3+cth1*sth2*salp2+sth1*cth2*calp1*salp2-cth1*cth2*sth3*salp3+sth1*sth2*calp1)*b);
dUman_3(8) = p_L3_x_l3*m_l3*g*((sth2*cth1*cth3+cth2*sth1*calp1+cth2*cth1*sth3*calp2+sth2*sth1*calp1)*a + (sth2*sth1*cth3-cth2*cth1*calp1+cth2*sth1*sth3*calp2-sth2*cth1*calp1*calp2)*b + (-cth2*cth3*salp1+sth2*sth3*salp1*calp2)*c)                                                                    + p_L3_y_l3*m_l3*g*((-cth2*cth1*salp2*salp3+sth2*sth1*calp1-sth2*cth1*sth3*calp3+cth2*sth1*calp1+cth2*cth1*cth3*calp2*calp3+sth2*sth1*calp1)*a + (-cth2*sth1*salp2*salp3-sth2*cth1*calp1-sth2*sth1*sth3*calp3-cth2*cth1*calp1+cth2*sth1*cth3*calp2*calp3-sth2*cth1*calp1)*b + (sth2*cth3*salp1*calp2*calp3+cth2*sth3*salp1*calp3-sth2*salp1*salp2*salp3)*c)                     + p_L3_z_l3*m_l3*g*((sth2*cth1*sth3*salp3+cth2*sth1*calp1-cth2*cth1*salp2*calp3+sth2*sth1*calp1-cth2*cth1*cth3*calp2*salp3+sth2*sth1*calp1)*a - (sth2*sth1*sth3*salp3-cth2*cth1*calp1-cth2*sth1*salp2*calp3-sth2*cth1*calp1-cth2*sth1*cth3*calp2*salp3-sth2*cth1*calp1)*b + (-cth2*sth3*salp1*salp3-sth2*salp1*salp2*calp3-sth2*cth3*salp1*calp2*salp3)*c);
dUman_3(9) = p_L3_x_l3*m_l3*g*((sth3*(cth1*cth2-sth1*sth2*calp1)+cth3*(cth1*sth2*calp2-sth1*salp1*salp2+sth1*cth2*calp1*calp2))*a + (sth3*(sth1*cth2+cth1*sth2*calp1)+cth3*(cth1*salp1*salp2+sth1*sth2*calp2-cth1*cth2*calp1*calp2))*b + (-cth3*(calp1*salp2+cth2*salp1*calp2)+sth3*sth2*salp1)*c)      + p_L3_y_l3*m_l3*g*((-sth3*calp3*(cth1*sth2*calp2-sth1*salp1*salp2+sth1*cth2*calp1*calp2-calp3*(cth1*cth2-sth1*sth2*calp1))*a + (-sth3*calp3*(cth1*salp1*salp2+sth1*sth2*calp2-cth1*cth2*calp1*calp2+cth3*calp3*(sth1*cth2+cth1*sth2*calp1)))*b + (-sth3*calp3*(calp1*salp2+cth2*salp1*calp2)+cth3*sth2*salp1*calp3))*c)                                                        + p_L3_z_l3*m_l3*g*((sth3*salp3*(cth1*sth2*calp2-sth1*salp1*salp2+sth1*cth2*calp1*calp2)-cth3*salp3*(cth1*cth2-sth1*sth2*calp1)))*a +(sth3*salp3*(cth1*salp1*salp2+sth1*sth2*calp2-cth1*cth2+calp1*calp2)-cth3*salp3*(sth1*cth2+cth1*sth2*calp1))*b + (-cth3*sth2*salp1*salp3-sth3*salp3*(calp1*salp2+cth2*salp1*calp2)*c);

G_est = dUuav + dUman_1 + dUman_2 + dUman_3;

== matlab function wrench_observer_R2016b/Wrench Observer Mom. based Method/Coriolis_Matrix/Coriolis_Matrix_simplified/MATLAB Function ==
  data: C11 input; C output; C12 input; C13 input; C21 input; C22 input; C23 input; C31 input; C32 input; C33 input
function C = Coriolis_Matrix(C11,C12,C13,C21,C22,C23,C31,C32,C33)
C = zeros(9);
C = [C11,C12,C13;C21,C22,C23;C31,C32,C33];

== matlab function wrench_observer_R2016b/Wrench Observer EKF/MATLAB Function ==
  settings: updateMethod=DISCRETE
  data: F input; xhatOut output; C input; meas input; yhatOut output; w_e_hat output; N_p parameter; N_m parameter
function [xhatOut,yhatOut,w_e_hat] = EKF(F,C,meas, N_p, N_m)
%% initialisation
persistent P xhat
if isempty(P)
    xhat = [1 0.75 1 0 0 0 0.1 0.1 0.1 0 0 0 pi/3 pi/3 pi/3 0 0 0 0 0 0 0 0 0 0 0 0 0 0 0 0 0 0 0 0 0]';
    P = zeros(36);
    % detect errors
    [m2,n2] = size(N_p);
    if ((m2 ~= 36) || (n2 ~= 36))
        fprintf('Error: Process covariance matrix has wrong dimensions. \n Expected a [36x36] matrix. \n The dimensions are [%dx%d].\n',m2,n2)
    end  
    [m3,n3] = size(N_m);
    if ((m3 ~= 27) || (n3 ~= 27))
        fprintf('Error: Measurement covariance matrix has wrong dimensions. \n Expected a [27x27] matrix. \n The dimensions are [%dx%d].\n',m2,n2)
    end  
    if any(any(isnan(N_p)))
        fprintf('Error: Process covariance matrix contains NaN values.\n')
    end
    if any(any(isnan(N_m)))
        fprintf('Error: Measurement covariance matrix contains NaN values.\n')
    end
end
%% loop
% detect errors
[m1,n1] = size(meas);
if ((m1 ~= 27) || (n1 ~= 1))
    fprintf('Error: Measurement vector has wrong dimensions. \n Expected a [27x1] vector. \n The dimensions are [%dx%d].\n',m1,n1)
end
if any(isnan(meas))
    fprintf('Error: Measurement vector contains NaN values.\n')
end
%% prediction
xhat = F*xhat;
P = F*P*F' + N_p;
% fprintf('P has NaN: %f \n',double(any(isnan(P(:)))))

%% Kalman gain
K = P*C'*inv(C*P*C'+N_m);

%% correction
xhat = xhat + K*(meas - C*xhat);
P = (eye(size(K,1)) - K*C)*P;

%% output
xhatOut = xhat;
yhatOut = C*xhatOut;
f_e_hat = xhat(22:24);
t_e_hat = xhat(28:30);
tman_e_hat = xhat(34:36);
w_e_hat = [f_e_hat' t_e_hat' tman_e_hat']';
